simulink model "simple_streaming_txrx"  (Simulink 6.6)
settings: Solver=ode45  StartTime=0.0  StopTime=inf  RelTol=1e-3
InitFcn:
  | simple_streaming_init
StartFcn:
  | simple_streaming_init
undefined symbols (not defined in the file): dmf, gcbh, get, modConstellation_qam16, modConstellation_qam64, modConstellation_qpsk, rcosfir, symbolRomLen, txLSFR_initValues, txLSFR_polynomials, viqAvgLen, xlBlockLoadCallback, xlGetSimulinkPeriod
libraries: xbsIndex_r4 x506, commchan3 x2, commsink2 x1
(part 4 of 5)

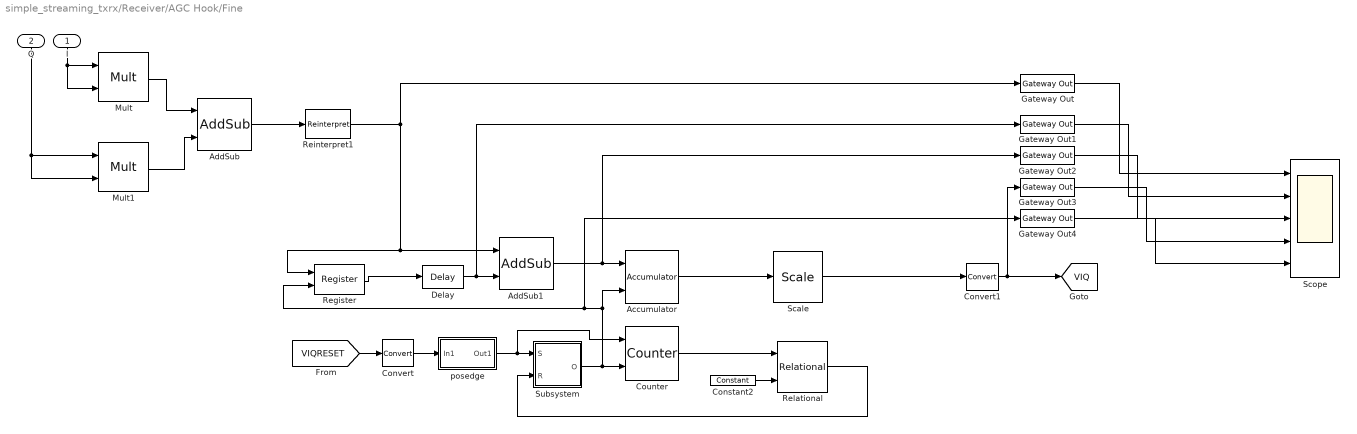
== system simple_streaming_txrx/Receiver/AGC Hook/Fine ==
  I : Inport  Orientation=down
  Q : Inport  Orientation=down  Port=2
  Accumulator : xbsIndex_r4/Accumulator  operation=Add  n_bits=30+ceil(log2(viqAvgLen))  overflow=Flag as error  scale=1  rst=on  hasbypass=off  en=off  dbl_ovrd=off  use_behavioral_HDL=on  block_type=accum
      settings: infoedit="Adder or subtractor-based accumulator.   Output type and binary point position match the input.<P><P>Hardware notes: When \"Reinitialize with input 'b' on reset\" is selected, the accumulator is forced to run at the system rate even if the input 'b' is running at a slower rate."  block_version=10.1.2
  AddSub : xbsIndex_r4/AddSub  mode=Addition  use_carryin=off  use_carryout=off  en=off  latency=0  precision=Full  arith_type=Unsigned  n_bits=16  bin_pt=14  quantization=Truncate  overflow=Wrap  dbl_ovrd=off  use_behavioral_HDL=off  pipelined=off  use_rpm=on  block_type=addsub
      settings: xl_area=[17 0 0 32 0 0 0]  block_version=10.1.2
  AddSub1 : xbsIndex_r4/AddSub  mode=Subtraction  use_carryin=off  use_carryout=off  en=off  latency=0  precision=Full  arith_type="Signed  (2's comp)"  n_bits=32  bin_pt=0  quantization=Truncate  overflow=Wrap  dbl_ovrd=off  use_behavioral_HDL=off  pipelined=off  use_rpm=on  block_type=addsub
      settings: block_version=10.1.2
  Constant2 : xbsIndex_r4/Constant  arith_type=Unsigned  const=viqAvgLen+2  n_bits=ceil(log2(viqAvgLen+1))  bin_pt=0  explicit_period=off  period=1  equ=P=C  opselect=C  inp2=PCIN>>17  opr=+  inp1=P  carry=CIN  dbl_ovrd=off  block_type=constant
      settings: block_version=10.1.2
  Convert : xbsIndex_r4/Convert  arith_type=Boolean  n_bits=16  bin_pt=14  quantization=Truncate  overflow=Wrap  latency=0  dbl_ovrd=off  pipeline=off  block_type=convert
      settings: block_version=10.1.2
  Convert1 : xbsIndex_r4/Convert  arith_type=Unsigned  n_bits=32  bin_pt=0  quantization=Truncate  overflow=Wrap  latency=0  dbl_ovrd=off  pipeline=off  block_type=convert
      settings: block_version=10.1.2
  Counter : xbsIndex_r4/Counter  cnt_type=Free Running  cnt_to=Inf  operation=Up  start_count=0  cnt_by_val=1  arith_type=Unsigned  n_bits=ceil(log2(viqAvgLen+1))  bin_pt=0  load_pin=off  rst=on  en=on  explicit_period=on  period=1/8  dbl_ovrd=off  use_behavioral_HDL=off  use_rpm=off  block_type=counter
      settings: block_version=10.1.2
  Delay : xbsIndex_r4/Delay  en=off  latency=viqAvgLen  dbl_ovrd=off  reg_retiming=off  block_type=delay
      settings: block_version=10.1.2
  Gateway Out{,1..4} (5 alike) : xbsIndex_r4/Gateway Out  hdl_port=off  timing_constraint=None  locs_specified=off  LOCs={}  block_type=gatewayout
      settings: infoedit="Gateway out block.  Converts Xilinx fixed point inputs into ouputs of type Simulink integer, double, or fixed point.<P><P>Hardware notes:  In hardware these blocks become top level output ports or are discarded, depending on how they are configured."  block_version=10.1.2
  Mult : xbsIndex_r4/Mult  precision=Full  arith_type=Unsigned  n_bits=32  bin_pt=32  quantization=Truncate  overflow=Saturate  en=off  latency=3  dbl_ovrd=off  use_behavioral_HDL=off  use_embedded=on  opt=Speed  optimum_pipeline=off  pipeline=on  use_rpm=on  placement_style=Triangular  block_type=mult
      settings: infoedit=Hardware notes: To use the internal pipeline stage of the dedicated multiplier you must select 'Pipeline for maximum performance'.  xl_area=[31 62 0 30 0 1 0]  block_version=10.1.2
  Mult1 : xbsIndex_r4/Mult  precision=Full  arith_type=Unsigned  n_bits=32  bin_pt=32  quantization=Truncate  overflow=Saturate  en=off  latency=3  dbl_ovrd=off  use_behavioral_HDL=off  use_embedded=on  opt=Speed  optimum_pipeline=off  pipeline=on  use_rpm=on  placement_style=Triangular  block_type=mult
      settings: infoedit=Hardware notes: To use the internal pipeline stage of the dedicated multiplier you must select 'Pipeline for maximum performance'.  xl_area=[31 62 0 30 0 1 0]  block_version=10.1.2
  Register : xbsIndex_r4/Register  init=0  rst=on  en=off  dbl_ovrd=off  block_type=register
      settings: block_version=10.1.2
  Reinterpret1 : xbsIndex_r4/Reinterpret  force_arith_type=on  arith_type=Unsigned  force_bin_pt=on  bin_pt=0  block_type=reinterpret
      settings: infoedit="Changes signal type without altering the binary representation.   You can changed the signal between signed and unsigned, and relocate the binary point.<P><P>Hardware notes: In hardware this block costs nothing.<P><P>Example:  Suppose the input is 6 bits wide, signed, with 2 fractional bits, and the output is forced to unsigned with 0 fractional bits.  Then an input of -2.0 (1110.00 in binary 2's complement) becomes an output of 56 (111000 in binary)."  block_version=10.1.2
  Relational : xbsIndex_r4/Relational  mode=a=b  en=off  latency=1  dbl_ovrd=off  block_type=relational
      settings: block_version=10.1.2
  Scale : xbsIndex_r4/Scale  scale_factor=-ceil(log2(viqAvgLen))  dbl_ovrd=off  block_type=scale
      settings: infoedit=Scales input by a power of two by adjusting the binary point position.<P><P>Hardware notes: In hardware this block costs nothing.  block_version=10.1.2
  Scope : Scope  NumInputPorts=5
      settings: YMin=0~0~-1.5e+006~1.06e+006~-1  YMax=2.75e+006~3e+006~2.5e+006~1.145e+006~1
  Subsystem : Subsystem
  posedge : Subsystem
  tag scope: VIQ=global
  wires:
  Mult1/1 -> AddSub/2
  Mult/1 -> AddSub/1
  I/1 -> Mult/1, Mult/2
  Q/1 -> Mult1/1, Mult1/2
  [VIQRESET] -> Convert/1
  posedge/1(Out1) -> Counter/1, Subsystem/1(S)
  Subsystem/1(O) -> Counter/2, Accumulator/2, Register/2, Gateway Out4/1
  Constant2/1 -> Relational/2
  Counter/1 -> Relational/1
  Relational/1 -> Subsystem/2(R)
  Accumulator/1 -> Scale/1
  Delay/1 -> AddSub1/2, Gateway Out1/1
  AddSub/1 -> Reinterpret1/1
  AddSub1/1 -> Accumulator/1, Gateway Out2/1
  Convert/1 -> posedge/1(In1)
  Convert1/1 -> [VIQ], Gateway Out3/1
  Reinterpret1/1 -> Gateway Out/1, AddSub1/1, Register/1
  Scale/1 -> Convert1/1
  Gateway Out/1 -> Scope/1
  Gateway Out1/1 -> Scope/2
  Gateway Out2/1 -> Scope/3
  Gateway Out3/1 -> Scope/4
  Gateway Out4/1 -> Scope/5
  Register/1 -> Delay/1

== system simple_streaming_txrx/Receiver/Carrier Recovery/2nd Order Filter ==
  Phase Error : Inport
  Reset : Inport  Port=2
  AddSub1 : xbsIndex_r4/AddSub  mode=Addition  use_carryin=off  use_carryout=off  en=off  latency=0  precision=Full  arith_type="Signed  (2's comp)"  n_bits=8  bin_pt=2  quantization=Truncate  overflow=Flag as error  dbl_ovrd=off  use_behavioral_HDL=on  pipelined=off  use_rpm=on  block_type=addsub
      settings: xl_area=[19 0 0 36 0 0 0]  block_version=10.1
  AddSub2 : xbsIndex_r4/AddSub  mode=Addition  use_carryin=off  use_carryout=off  en=off  latency=0  precision=User Defined  arith_type="Signed  (2's comp)"  n_bits=35  bin_pt=34  quantization=Truncate  overflow=Flag as error  dbl_ovrd=off  use_behavioral_HDL=on  pipelined=off  use_rpm=on  block_type=addsub
      settings: xl_area=[19 0 0 36 0 0 0]  block_version=10.1
  Delay1 : xbsIndex_r4/Delay  en=off  latency=1  dbl_ovrd=off  reg_retiming=off  block_type=delay
      settings: xl_area=[18 35 0 0 0 0 0]  block_version=10.1
  Delay2 : xbsIndex_r4/Delay  en=off  latency=1  dbl_ovrd=off  reg_retiming=off  block_type=delay
      settings: xl_area=[18 35 0 0 0 0 0]  block_version=10.1
  Mult1 : xbsIndex_r4/Mult  precision=User Defined  arith_type="Signed  (2's comp)"  n_bits=35  bin_pt=34  quantization=Truncate  overflow=Flag as error  en=off  latency=3  dbl_ovrd=off  use_behavioral_HDL=off  use_embedded=on  opt=Speed  optimum_pipeline=off  pipeline=on  use_rpm=on  placement_style=Rectangular shape  block_type=mult
      settings: infoedit=Hardware notes: To use the internal pipeline stage of the dedicated multiplier you must select 'Pipeline for maximum performance'.  xl_area=[89 143 0 153 0 4 0]  block_version=10.1
  Mult2 : xbsIndex_r4/Mult  precision=User Defined  arith_type="Signed  (2's comp)"  n_bits=35  bin_pt=34  quantization=Truncate  overflow=Flag as error  en=off  latency=3  dbl_ovrd=off  use_behavioral_HDL=off  use_embedded=on  opt=Speed  optimum_pipeline=off  pipeline=on  use_rpm=on  placement_style=Rectangular shape  block_type=mult
      settings: infoedit=Hardware notes: To use the internal pipeline stage of the dedicated multiplier you must select 'Pipeline for maximum performance'.  xl_area=[89 143 0 153 0 4 0]  block_version=10.1
  Register1 : xbsIndex_r4/Register  init=0  rst=on  en=off  dbl_ovrd=off  block_type=register
      settings: xl_area=[18 36 0 0 0 0 0]  block_version=10.1
  Register2 : xbsIndex_r4/Register  Orientation=left  init=0  rst=on  en=off  dbl_ovrd=off  block_type=register
      settings: xl_area=[18 35 0 0 0 0 0]  block_version=10.1
  Phase Inc : Outport
  wires:
  Delay2/1 -> AddSub1/1
  Register2/1 -> AddSub2/2
  AddSub2/1 -> Delay1/1, Register2/1
  Mult1/1 -> AddSub2/1
  Mult2/1 -> Delay2/1
  AddSub1/1 -> Register1/1
  Reset/1 -> Register1/2, Register2/2
  Register1/1 -> Phase Inc/1
  Phase Error/1 -> Mult2/2, Mult1/1
  [CFO_KI] -> Mult1/2
  [CFO_KP] -> Mult2/1
  Delay1/1 -> AddSub1/2

== system simple_streaming_txrx/Receiver/Carrier Recovery/Phase Error Detector ==
  I : Inport
  Q : Inport  Port=2
  AddSub : xbsIndex_r4/AddSub  mode=Subtraction  use_carryin=off  use_carryout=off  en=off  latency=0  precision=Full  arith_type="Signed  (2's comp)"  n_bits=16  bin_pt=13  quantization=Truncate  overflow=Wrap  dbl_ovrd=off  use_behavioral_HDL=on  pipelined=off  use_rpm=on  block_type=addsub
      settings: xl_area=[10 0 0 19 0 0 0]  block_version=10.1
  Mult : xbsIndex_r4/Mult  precision=Full  arith_type="Signed  (2's comp)"  n_bits=16  bin_pt=14  quantization=Truncate  overflow=Wrap  en=off  latency=1  dbl_ovrd=off  use_behavioral_HDL=off  use_embedded=on  opt=Speed  optimum_pipeline=off  pipeline=on  use_rpm=on  placement_style=Rectangular shape  block_type=mult
      settings: infoedit=Hardware notes: To use the internal pipeline stage of the dedicated multiplier you must select 'Pipeline for maximum performance'.  xl_area=[9 0 0 18 0 1 0]  block_version=10.1
  Mult1 : xbsIndex_r4/Mult  precision=Full  arith_type="Signed  (2's comp)"  n_bits=16  bin_pt=14  quantization=Truncate  overflow=Wrap  en=off  latency=1  dbl_ovrd=off  use_behavioral_HDL=off  use_embedded=on  opt=Speed  optimum_pipeline=off  pipeline=on  use_rpm=on  placement_style=Rectangular shape  block_type=mult
      settings: infoedit=Hardware notes: To use the internal pipeline stage of the dedicated multiplier you must select 'Pipeline for maximum performance'.  xl_area=[9 0 0 18 0 1 0]  block_version=10.1
  Threshold : xbsIndex_r4/Threshold  en=off  latency=0  dbl_ovrd=off  block_type=sgn
      settings: infoedit="Presents -1 as output if input is negative; otherwise presents 1.  Output is a two bit signed number."  xl_area=[0 0 0 0 0 0 0]  block_version=10.1
  Threshold1 : xbsIndex_r4/Threshold  en=off  latency=0  dbl_ovrd=off  block_type=sgn
      settings: infoedit="Presents -1 as output if input is negative; otherwise presents 1.  Output is a two bit signed number."  xl_area=[0 0 0 0 0 0 0]  block_version=10.1
  Err : Outport
  wires:
  Threshold1/1 -> Mult1/1
  Threshold/1 -> Mult/1
  Mult/1 -> AddSub/1
  Mult1/1 -> AddSub/2
  I/1 -> Mult1/2, Threshold/1
  Q/1 -> Mult/2, Threshold1/1
  AddSub/1 -> Err/1

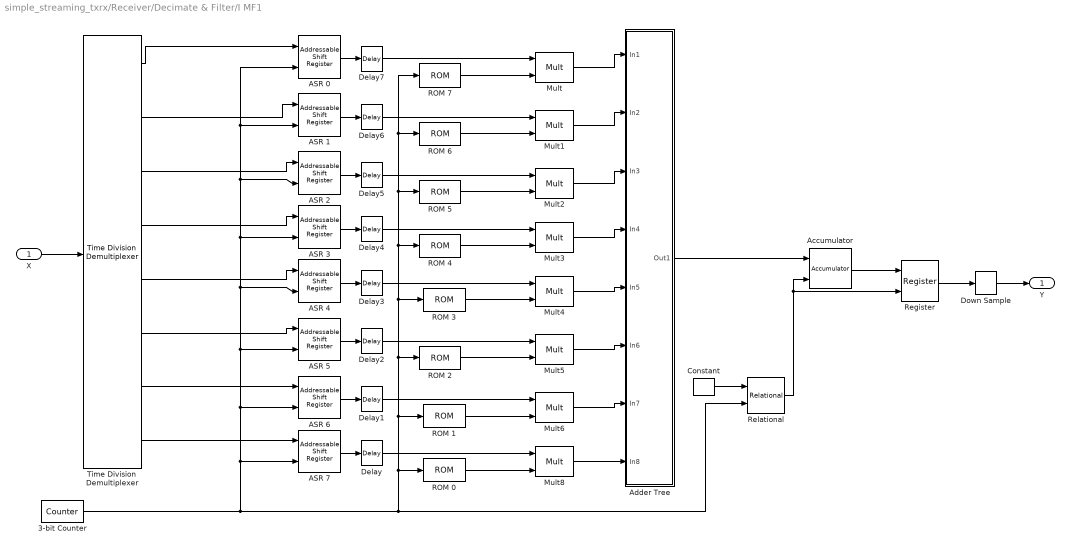
== system simple_streaming_txrx/Receiver/Decimate & Filter/I MF1 ==
  X : Inport
  3-bit Counter : xbsIndex_r4/Counter  cnt_type=Free Running  cnt_to=Inf  operation=Up  start_count=0  cnt_by_val=1  arith_type=Unsigned  n_bits=3  bin_pt=0  load_pin=off  rst=off  en=off  explicit_period=off  period=data_samplePeriod  dbl_ovrd=off  use_behavioral_HDL=off  use_rpm=on  block_type=counter
      settings: xl_area=[3 3 0 3 0 0 0]  block_version=10.1
  ASR {0..7} (8 alike) : xbsIndex_r4/Addressable Shift Register  infer_latency=on  depth=2  initVector=[0]  en=off  dbl_ovrd=off  use_behavioral_HDL=off  use_rpm=on  block_type=addrsr
      settings: infoedit="Delay of configurable length.  Any element in the delay line can be addressed and driven onto the output port.<br><br>Hardware notes: Implemented using SRL16s.  If Virtex-4, Virtex-II or Spartan-3 devices are used, multiple SRLC16s are cascaded together."  xl_area=[9 0 0 18 0 0 0]  block_version=10.1
  Accumulator : xbsIndex_r4/Accumulator  operation=Add  n_bits=add_prec  overflow=Wrap  scale=1  rst=on  hasbypass=on  en=off  dbl_ovrd=off  use_behavioral_HDL=on  block_type=accum
      settings: infoedit="Adder or subtractor-based accumulator.   Output type and binary point position match the input.<P><P>Hardware notes: When \"Reinitialize with input 'b' on reset\" is selected, the accumulator is forced to run at the system rate even if the input 'b' is running at a slower rate."  xl_area=[9 17 0 16 0 0 0]  block_version=10.1
  Adder Tree : Subsystem
  Constant : xbsIndex_r4/Constant  arith_type=Unsigned  const=3  n_bits=3  bin_pt=0  explicit_period=on  period=data_samplePeriod  equ=P=C  opselect=C  inp2=PCIN>>17  opr=+  inp1=P  carry=CIN  dbl_ovrd=off  block_type=constant
      settings: block_version=10.1
  Delay{,1..7} (8 alike) : xbsIndex_r4/Delay  en=off  latency=1  dbl_ovrd=off  reg_retiming=off  block_type=delay
      settings: xl_area=[9 18 0 0 0 0 0]  block_version=10.1
  Down Sample : xbsIndex_r4/Down Sample  sample_ratio=8  sample_phase=First Value of Frame  en=off  latency=0  dbl_ovrd=off  block_type=dsamp
      settings: xl_area=[17 17 0 16 0 0 0]  block_version=10.1
  Mult{,1..6,8} (8 alike) : xbsIndex_r4/Mult  precision=User Defined  arith_type="Signed  (2's comp)"  n_bits=mult_prec  bin_pt=mult_bp  quantization=Truncate  overflow=Flag as error  en=off  latency=multLatency  dbl_ovrd=off  use_behavioral_HDL=off  use_embedded=on  opt=Speed  optimum_pipeline=off  pipeline=on  use_rpm=on  placement_style=Rectangular shape  block_type=mult
      settings: infoedit=Hardware notes: To use the internal pipeline stage of the dedicated multiplier you must select 'Pipeline for maximum performance'.  xl_area=[9 -13 0 18 0 1 0]  block_version=10.1
  ROM 0 : xbsIndex_r4/ROM  depth=polyphaseBranches  initVector=h(1:subFilterLength)  distributed_mem=Distributed memory  rst=off  init_reg=0  en=off  latency=1  arith_type="Signed  (2's comp)"  n_bits=coeff_prec  bin_pt=coeff_bp  dbl_ovrd=off  optimize=Area  use_rpm=off  block_type=sprom
      settings: xl_area=[7 14 0 13 0 0 0]  block_version=10.1
  ROM 1 : xbsIndex_r4/ROM  depth=polyphaseBranches  initVector=h(1*subFilterLength+1:2*subFilterLength)  distributed_mem=Distributed memory  rst=off  init_reg=0  en=off  latency=1  arith_type="Signed  (2's comp)"  n_bits=coeff_prec  bin_pt=coeff_bp  dbl_ovrd=off  optimize=Area  use_rpm=off  block_type=sprom
      settings: xl_area=[7 14 0 14 0 0 0]  block_version=10.1
  ROM 2 : xbsIndex_r4/ROM  depth=polyphaseBranches  initVector=h(2*subFilterLength+1:3*subFilterLength)  distributed_mem=Distributed memory  rst=off  init_reg=0  en=off  latency=1  arith_type="Signed  (2's comp)"  n_bits=coeff_prec  bin_pt=coeff_bp  dbl_ovrd=off  optimize=Area  use_rpm=off  block_type=sprom
      settings: xl_area=[7 14 0 14 0 0 0]  block_version=10.1
  ROM 3 : xbsIndex_r4/ROM  depth=polyphaseBranches  initVector=h(3*subFilterLength+1:4*subFilterLength)  distributed_mem=Distributed memory  rst=off  init_reg=0  en=off  latency=1  arith_type="Signed  (2's comp)"  n_bits=coeff_prec  bin_pt=coeff_bp  dbl_ovrd=off  optimize=Area  use_rpm=off  block_type=sprom
      settings: xl_area=[7 14 0 14 0 0 0]  block_version=10.1
  ROM 4 : xbsIndex_r4/ROM  depth=polyphaseBranches  initVector=h(4*subFilterLength+1:5*subFilterLength)  distributed_mem=Distributed memory  rst=off  init_reg=0  en=off  latency=1  arith_type="Signed  (2's comp)"  n_bits=coeff_prec  bin_pt=coeff_bp  dbl_ovrd=off  optimize=Area  use_rpm=off  block_type=sprom
      settings: xl_area=[7 14 0 14 0 0 0]  block_version=10.1
  ROM 5 : xbsIndex_r4/ROM  depth=polyphaseBranches  initVector=h(5*subFilterLength+1:6*subFilterLength)  distributed_mem=Distributed memory  rst=off  init_reg=0  en=off  latency=1  arith_type="Signed  (2's comp)"  n_bits=coeff_prec  bin_pt=coeff_bp  dbl_ovrd=off  optimize=Area  use_rpm=off  block_type=sprom
      settings: xl_area=[7 14 0 14 0 0 0]  block_version=10.1
  ROM 6 : xbsIndex_r4/ROM  depth=polyphaseBranches  initVector=h(6*subFilterLength+1:7*subFilterLength)  distributed_mem=Distributed memory  rst=off  init_reg=0  en=off  latency=1  arith_type="Signed  (2's comp)"  n_bits=coeff_prec  bin_pt=coeff_bp  dbl_ovrd=off  optimize=Area  use_rpm=off  block_type=sprom
      settings: xl_area=[7 14 0 14 0 0 0]  block_version=10.1
  ROM 7 : xbsIndex_r4/ROM  depth=polyphaseBranches  initVector=h(7*subFilterLength+1:8*subFilterLength)  distributed_mem=Distributed memory  rst=off  init_reg=0  en=off  latency=1  arith_type="Signed  (2's comp)"  n_bits=coeff_prec  bin_pt=coeff_bp  dbl_ovrd=off  optimize=Area  use_rpm=off  block_type=sprom
      settings: xl_area=[7 14 0 14 0 0 0]  block_version=10.1
  Register : xbsIndex_r4/Register  init=0  rst=off  en=on  dbl_ovrd=off  block_type=register
      settings: xl_area=[8 16 0 0 0 0 0]  block_version=10.1
  Relational : xbsIndex_r4/Relational  mode=a=b  en=off  latency=0  dbl_ovrd=off  block_type=relational
      settings: xl_area=[1 0 0 2 0 0 0]  block_version=10.1
  Time Division Demultiplexer : xbsIndex_r4/Time Division Demultiplexer  frame_pattern=ones(1,8)  impl_style=Multiple Channel  vin=off  dbl_ovrd=off  explicit_period=off  period=1  block_type=tdd
      settings: infoedit=Samples presented at the input are selected and down-sampled according to the frame sampling pattern specified. The sampled input is presented either as a single or multiple channel at the output.  xl_area=[135 270 0 0 0 0 0]  block_version=10.1
  Y : Outport
  wires:
  3-bit Counter/1 -> ROM 6/1, ROM 7/1, ROM 5/1, ROM 4/1, ROM 3/1, ROM 2/1, ROM 1/1, ROM 0/1, Relational/2, ASR 7/2, ASR 6/2, ASR 5/2, ASR 4/2, ASR 3/2, ASR 2/2, ASR 0/2, ASR 1/2
  ASR 7/1 -> Delay/1
  ASR 6/1 -> Delay1/1
  ASR 5/1 -> Delay2/1
  ASR 4/1 -> Delay3/1
  ASR 3/1 -> Delay4/1
  ASR 2/1 -> Delay5/1
  ASR 1/1 -> Delay6/1
  ASR 0/1 -> Delay7/1
  Mult8/1 -> Adder Tree/8(In8)
  Mult6/1 -> Adder Tree/7(In7)
  Mult5/1 -> Adder Tree/6(In6)
  Mult4/1 -> Adder Tree/5(In5)
  Mult3/1 -> Adder Tree/4(In4)
  Mult2/1 -> Adder Tree/3(In3)
  Mult1/1 -> Adder Tree/2(In2)
  Mult/1 -> Adder Tree/1(In1)
  ROM 0/1 -> Mult8/2
  ROM 1/1 -> Mult6/2
  ROM 2/1 -> Mult5/2
  ROM 3/1 -> Mult4/2
  ROM 4/1 -> Mult3/2
  ROM 5/1 -> Mult2/2
  ROM 6/1 -> Mult1/2
  ROM 7/1 -> Mult/2
  Accumulator/1 -> Register/1
  Constant/1 -> Relational/1
  Relational/1 -> Accumulator/2, Register/2
  Down Sample/1 -> Y/1
  Register/1 -> Down Sample/1
  Adder Tree/1(Out1) -> Accumulator/1
  X/1 -> Time Division Demultiplexer/1
  Time Division Demultiplexer/1 -> ASR 0/1
  Time Division Demultiplexer/2 -> ASR 1/1
  Time Division Demultiplexer/3 -> ASR 2/1
  Time Division Demultiplexer/4 -> ASR 3/1
  Time Division Demultiplexer/5 -> ASR 4/1
  Time Division Demultiplexer/6 -> ASR 5/1
  Time Division Demultiplexer/7 -> ASR 6/1
  Time Division Demultiplexer/8 -> ASR 7/1
  Delay/1 -> Mult8/1
  Delay1/1 -> Mult6/1
  Delay2/1 -> Mult5/1
  Delay3/1 -> Mult4/1
  Delay4/1 -> Mult3/1
  Delay5/1 -> Mult2/1
  Delay6/1 -> Mult1/1
  Delay7/1 -> Mult/1

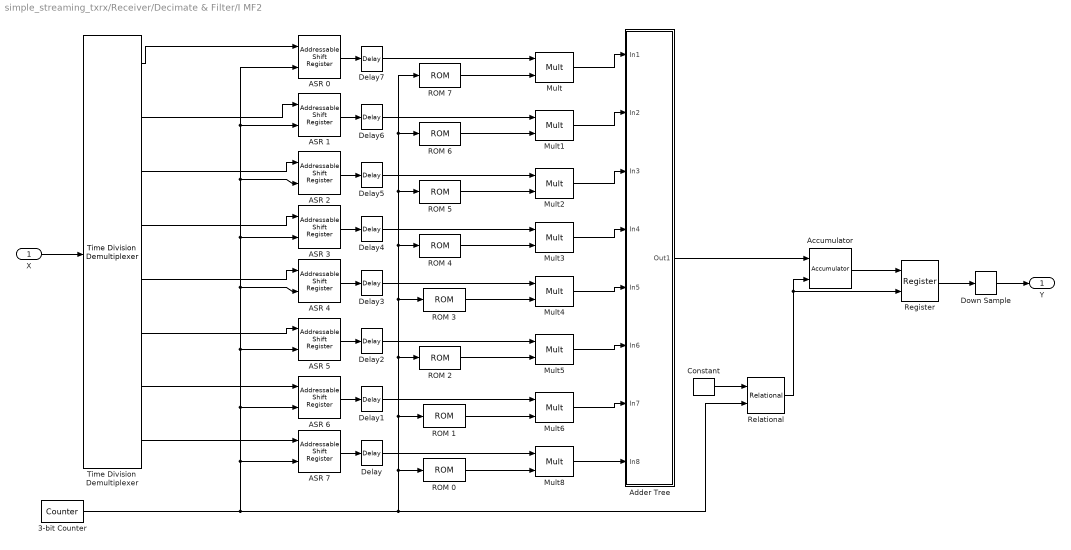
== system simple_streaming_txrx/Receiver/Decimate & Filter/I MF2 ==
  X : Inport
  3-bit Counter : xbsIndex_r4/Counter  cnt_type=Free Running  cnt_to=Inf  operation=Up  start_count=0  cnt_by_val=1  arith_type=Unsigned  n_bits=3  bin_pt=0  load_pin=off  rst=off  en=off  explicit_period=off  period=data_samplePeriod  dbl_ovrd=off  use_behavioral_HDL=off  use_rpm=on  block_type=counter
      settings: xl_area=[3 3 0 3 0 0 0]  block_version=10.1
  ASR {0..7} (8 alike) : xbsIndex_r4/Addressable Shift Register  infer_latency=on  depth=2  initVector=[0]  en=off  dbl_ovrd=off  use_behavioral_HDL=off  use_rpm=on  block_type=addrsr
      settings: infoedit="Delay of configurable length.  Any element in the delay line can be addressed and driven onto the output port.<br><br>Hardware notes: Implemented using SRL16s.  If Virtex-4, Virtex-II or Spartan-3 devices are used, multiple SRLC16s are cascaded together."  xl_area=[9 0 0 18 0 0 0]  block_version=10.1
  Accumulator : xbsIndex_r4/Accumulator  operation=Add  n_bits=add_prec  overflow=Wrap  scale=1  rst=on  hasbypass=on  en=off  dbl_ovrd=off  use_behavioral_HDL=on  block_type=accum
      settings: infoedit="Adder or subtractor-based accumulator.   Output type and binary point position match the input.<P><P>Hardware notes: When \"Reinitialize with input 'b' on reset\" is selected, the accumulator is forced to run at the system rate even if the input 'b' is running at a slower rate."  xl_area=[9 17 0 16 0 0 0]  block_version=10.1
  Adder Tree : Subsystem
  Constant : xbsIndex_r4/Constant  arith_type=Unsigned  const=3  n_bits=3  bin_pt=0  explicit_period=on  period=data_samplePeriod  equ=P=C  opselect=C  inp2=PCIN>>17  opr=+  inp1=P  carry=CIN  dbl_ovrd=off  block_type=constant
      settings: block_version=10.1
  Delay{,1..7} (8 alike) : xbsIndex_r4/Delay  en=off  latency=1  dbl_ovrd=off  reg_retiming=off  block_type=delay
      settings: xl_area=[9 18 0 0 0 0 0]  block_version=10.1
  Down Sample : xbsIndex_r4/Down Sample  sample_ratio=8  sample_phase=First Value of Frame  en=off  latency=0  dbl_ovrd=off  block_type=dsamp
      settings: xl_area=[17 17 0 16 0 0 0]  block_version=10.1
  Mult{,1..6,8} (8 alike) : xbsIndex_r4/Mult  precision=User Defined  arith_type="Signed  (2's comp)"  n_bits=mult_prec  bin_pt=mult_bp  quantization=Truncate  overflow=Flag as error  en=off  latency=multLatency  dbl_ovrd=off  use_behavioral_HDL=off  use_embedded=on  opt=Speed  optimum_pipeline=off  pipeline=on  use_rpm=on  placement_style=Rectangular shape  block_type=mult
      settings: infoedit=Hardware notes: To use the internal pipeline stage of the dedicated multiplier you must select 'Pipeline for maximum performance'.  xl_area=[9 -13 0 18 0 1 0]  block_version=10.1
  ROM 0 : xbsIndex_r4/ROM  depth=polyphaseBranches  initVector=h(1:subFilterLength)  distributed_mem=Distributed memory  rst=off  init_reg=0  en=off  latency=1  arith_type="Signed  (2's comp)"  n_bits=coeff_prec  bin_pt=coeff_bp  dbl_ovrd=off  optimize=Area  use_rpm=off  block_type=sprom
      settings: xl_area=[7 14 0 13 0 0 0]  block_version=10.1
  ROM 1 : xbsIndex_r4/ROM  depth=polyphaseBranches  initVector=h(1*subFilterLength+1:2*subFilterLength)  distributed_mem=Distributed memory  rst=off  init_reg=0  en=off  latency=1  arith_type="Signed  (2's comp)"  n_bits=coeff_prec  bin_pt=coeff_bp  dbl_ovrd=off  optimize=Area  use_rpm=off  block_type=sprom
      settings: xl_area=[7 14 0 14 0 0 0]  block_version=10.1
  ROM 2 : xbsIndex_r4/ROM  depth=polyphaseBranches  initVector=h(2*subFilterLength+1:3*subFilterLength)  distributed_mem=Distributed memory  rst=off  init_reg=0  en=off  latency=1  arith_type="Signed  (2's comp)"  n_bits=coeff_prec  bin_pt=coeff_bp  dbl_ovrd=off  optimize=Area  use_rpm=off  block_type=sprom
      settings: xl_area=[7 14 0 14 0 0 0]  block_version=10.1
  ROM 3 : xbsIndex_r4/ROM  depth=polyphaseBranches  initVector=h(3*subFilterLength+1:4*subFilterLength)  distributed_mem=Distributed memory  rst=off  init_reg=0  en=off  latency=1  arith_type="Signed  (2's comp)"  n_bits=coeff_prec  bin_pt=coeff_bp  dbl_ovrd=off  optimize=Area  use_rpm=off  block_type=sprom
      settings: xl_area=[7 14 0 14 0 0 0]  block_version=10.1
  ROM 4 : xbsIndex_r4/ROM  depth=polyphaseBranches  initVector=h(4*subFilterLength+1:5*subFilterLength)  distributed_mem=Distributed memory  rst=off  init_reg=0  en=off  latency=1  arith_type="Signed  (2's comp)"  n_bits=coeff_prec  bin_pt=coeff_bp  dbl_ovrd=off  optimize=Area  use_rpm=off  block_type=sprom
      settings: xl_area=[7 14 0 14 0 0 0]  block_version=10.1
  ROM 5 : xbsIndex_r4/ROM  depth=polyphaseBranches  initVector=h(5*subFilterLength+1:6*subFilterLength)  distributed_mem=Distributed memory  rst=off  init_reg=0  en=off  latency=1  arith_type="Signed  (2's comp)"  n_bits=coeff_prec  bin_pt=coeff_bp  dbl_ovrd=off  optimize=Area  use_rpm=off  block_type=sprom
      settings: xl_area=[7 14 0 14 0 0 0]  block_version=10.1
  ROM 6 : xbsIndex_r4/ROM  depth=polyphaseBranches  initVector=h(6*subFilterLength+1:7*subFilterLength)  distributed_mem=Distributed memory  rst=off  init_reg=0  en=off  latency=1  arith_type="Signed  (2's comp)"  n_bits=coeff_prec  bin_pt=coeff_bp  dbl_ovrd=off  optimize=Area  use_rpm=off  block_type=sprom
      settings: xl_area=[7 14 0 14 0 0 0]  block_version=10.1
  ROM 7 : xbsIndex_r4/ROM  depth=polyphaseBranches  initVector=h(7*subFilterLength+1:8*subFilterLength)  distributed_mem=Distributed memory  rst=off  init_reg=0  en=off  latency=1  arith_type="Signed  (2's comp)"  n_bits=coeff_prec  bin_pt=coeff_bp  dbl_ovrd=off  optimize=Area  use_rpm=off  block_type=sprom
      settings: xl_area=[7 14 0 14 0 0 0]  block_version=10.1
  Register : xbsIndex_r4/Register  init=0  rst=off  en=on  dbl_ovrd=off  block_type=register
      settings: xl_area=[8 16 0 0 0 0 0]  block_version=10.1
  Relational : xbsIndex_r4/Relational  mode=a=b  en=off  latency=0  dbl_ovrd=off  block_type=relational
      settings: xl_area=[1 0 0 2 0 0 0]  block_version=10.1
  Time Division Demultiplexer : xbsIndex_r4/Time Division Demultiplexer  frame_pattern=ones(1,8)  impl_style=Multiple Channel  vin=off  dbl_ovrd=off  explicit_period=off  period=1  block_type=tdd
      settings: infoedit=Samples presented at the input are selected and down-sampled according to the frame sampling pattern specified. The sampled input is presented either as a single or multiple channel at the output.  xl_area=[135 270 0 0 0 0 0]  block_version=10.1
  Y : Outport
  wires:
  Delay7/1 -> Mult/1
  Delay6/1 -> Mult1/1
  Delay5/1 -> Mult2/1
  Delay4/1 -> Mult3/1
  Delay3/1 -> Mult4/1
  Delay2/1 -> Mult5/1
  Delay1/1 -> Mult6/1
  Delay/1 -> Mult8/1
  Time Division Demultiplexer/8 -> ASR 7/1
  Time Division Demultiplexer/7 -> ASR 6/1
  Time Division Demultiplexer/6 -> ASR 5/1
  Time Division Demultiplexer/5 -> ASR 4/1
  Time Division Demultiplexer/4 -> ASR 3/1
  Time Division Demultiplexer/3 -> ASR 2/1
  Time Division Demultiplexer/2 -> ASR 1/1
  Time Division Demultiplexer/1 -> ASR 0/1
  X/1 -> Time Division Demultiplexer/1
  Adder Tree/1(Out1) -> Accumulator/1
  Register/1 -> Down Sample/1
  Down Sample/1 -> Y/1
  Relational/1 -> Register/2, Accumulator/2
  Constant/1 -> Relational/1
  Accumulator/1 -> Register/1
  ROM 7/1 -> Mult/2
  ROM 6/1 -> Mult1/2
  ROM 5/1 -> Mult2/2
  ROM 4/1 -> Mult3/2
  ROM 3/1 -> Mult4/2
  ROM 2/1 -> Mult5/2
  ROM 1/1 -> Mult6/2
  ROM 0/1 -> Mult8/2
  Mult/1 -> Adder Tree/1(In1)
  Mult1/1 -> Adder Tree/2(In2)
  Mult2/1 -> Adder Tree/3(In3)
  Mult3/1 -> Adder Tree/4(In4)
  Mult4/1 -> Adder Tree/5(In5)
  Mult5/1 -> Adder Tree/6(In6)
  Mult6/1 -> Adder Tree/7(In7)
  Mult8/1 -> Adder Tree/8(In8)
  ASR 0/1 -> Delay7/1
  ASR 1/1 -> Delay6/1
  ASR 2/1 -> Delay5/1
  ASR 3/1 -> Delay4/1
  ASR 4/1 -> Delay3/1
  ASR 5/1 -> Delay2/1
  ASR 6/1 -> Delay1/1
  ASR 7/1 -> Delay/1
  3-bit Counter/1 -> ASR 1/2, ASR 0/2, ASR 2/2, ASR 3/2, ASR 4/2, ASR 5/2, ASR 6/2, ASR 7/2, Relational/2, ROM 0/1, ROM 1/1, ROM 2/1, ROM 3/1, ROM 4/1, ROM 5/1, ROM 7/1, ROM 6/1

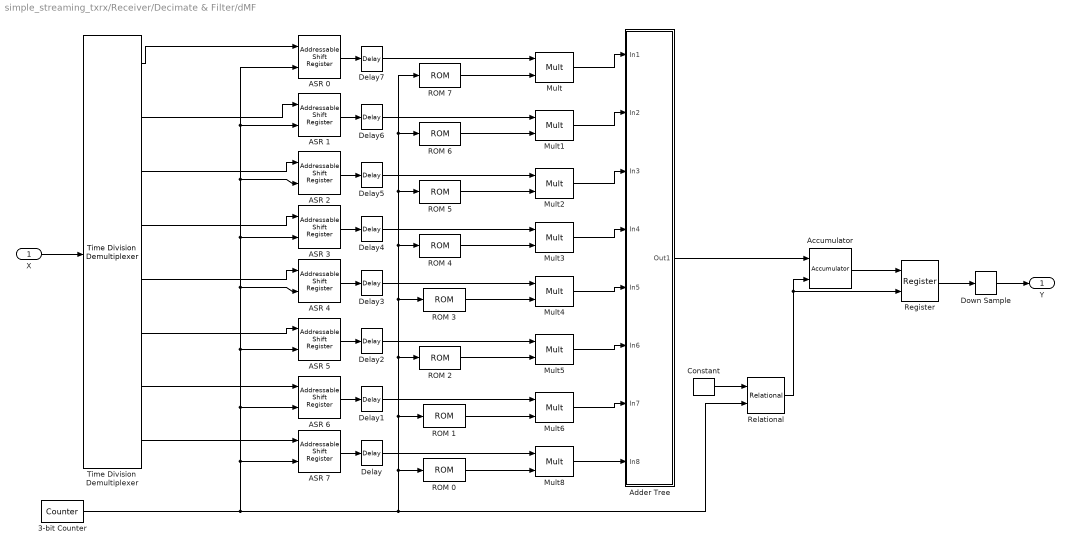
== system simple_streaming_txrx/Receiver/Decimate & Filter/dMF ==
  X : Inport
  3-bit Counter : xbsIndex_r4/Counter  cnt_type=Free Running  cnt_to=Inf  operation=Up  start_count=0  cnt_by_val=1  arith_type=Unsigned  n_bits=3  bin_pt=0  load_pin=off  rst=off  en=off  explicit_period=off  period=data_samplePeriod  dbl_ovrd=off  use_behavioral_HDL=off  use_rpm=on  block_type=counter
      settings: xl_area=[3 3 0 3 0 0 0]  block_version=10.1
  ASR {0..7} (8 alike) : xbsIndex_r4/Addressable Shift Register  infer_latency=on  depth=2  initVector=[0]  en=off  dbl_ovrd=off  use_behavioral_HDL=off  use_rpm=on  block_type=addrsr
      settings: infoedit="Delay of configurable length.  Any element in the delay line can be addressed and driven onto the output port.<br><br>Hardware notes: Implemented using SRL16s.  If Virtex-4, Virtex-II or Spartan-3 devices are used, multiple SRLC16s are cascaded together."  xl_area=[9 0 0 18 0 0 0]  block_version=10.1
  Accumulator : xbsIndex_r4/Accumulator  operation=Add  n_bits=add_prec  overflow=Wrap  scale=1  rst=on  hasbypass=on  en=off  dbl_ovrd=off  use_behavioral_HDL=on  block_type=accum
      settings: infoedit="Adder or subtractor-based accumulator.   Output type and binary point position match the input.<P><P>Hardware notes: When \"Reinitialize with input 'b' on reset\" is selected, the accumulator is forced to run at the system rate even if the input 'b' is running at a slower rate."  xl_area=[9 17 0 16 0 0 0]  block_version=10.1
  Adder Tree : Subsystem
  Constant : xbsIndex_r4/Constant  arith_type=Unsigned  const=3  n_bits=3  bin_pt=0  explicit_period=on  period=data_samplePeriod  equ=P=C  opselect=C  inp2=PCIN>>17  opr=+  inp1=P  carry=CIN  dbl_ovrd=off  block_type=constant
      settings: block_version=10.1
  Delay{,1..7} (8 alike) : xbsIndex_r4/Delay  en=off  latency=1  dbl_ovrd=off  reg_retiming=off  block_type=delay
      settings: xl_area=[9 18 0 0 0 0 0]  block_version=10.1
  Down Sample : xbsIndex_r4/Down Sample  sample_ratio=8  sample_phase=First Value of Frame  en=off  latency=0  dbl_ovrd=off  block_type=dsamp
      settings: xl_area=[17 17 0 16 0 0 0]  block_version=10.1
  Mult{,1..6,8} (8 alike) : xbsIndex_r4/Mult  precision=User Defined  arith_type="Signed  (2's comp)"  n_bits=mult_prec  bin_pt=mult_bp  quantization=Truncate  overflow=Flag as error  en=off  latency=multLatency  dbl_ovrd=off  use_behavioral_HDL=off  use_embedded=on  opt=Speed  optimum_pipeline=off  pipeline=on  use_rpm=on  placement_style=Rectangular shape  block_type=mult
      settings: infoedit=Hardware notes: To use the internal pipeline stage of the dedicated multiplier you must select 'Pipeline for maximum performance'.  xl_area=[9 -13 0 18 0 1 0]  block_version=10.1
  ROM 0 : xbsIndex_r4/ROM  depth=polyphaseBranches  initVector=h(1:subFilterLength)  distributed_mem=Distributed memory  rst=off  init_reg=0  en=off  latency=1  arith_type="Signed  (2's comp)"  n_bits=coeff_prec  bin_pt=coeff_bp  dbl_ovrd=off  optimize=Area  use_rpm=off  block_type=sprom
      settings: xl_area=[7 14 0 14 0 0 0]  block_version=10.1
  ROM 1 : xbsIndex_r4/ROM  depth=polyphaseBranches  initVector=h(1*subFilterLength+1:2*subFilterLength)  distributed_mem=Distributed memory  rst=off  init_reg=0  en=off  latency=1  arith_type="Signed  (2's comp)"  n_bits=coeff_prec  bin_pt=coeff_bp  dbl_ovrd=off  optimize=Area  use_rpm=off  block_type=sprom
      settings: xl_area=[7 14 0 14 0 0 0]  block_version=10.1
  ROM 2 : xbsIndex_r4/ROM  depth=polyphaseBranches  initVector=h(2*subFilterLength+1:3*subFilterLength)  distributed_mem=Distributed memory  rst=off  init_reg=0  en=off  latency=1  arith_type="Signed  (2's comp)"  n_bits=coeff_prec  bin_pt=coeff_bp  dbl_ovrd=off  optimize=Area  use_rpm=off  block_type=sprom
      settings: xl_area=[7 14 0 14 0 0 0]  block_version=10.1
  ROM 3 : xbsIndex_r4/ROM  depth=polyphaseBranches  initVector=h(3*subFilterLength+1:4*subFilterLength)  distributed_mem=Distributed memory  rst=off  init_reg=0  en=off  latency=1  arith_type="Signed  (2's comp)"  n_bits=coeff_prec  bin_pt=coeff_bp  dbl_ovrd=off  optimize=Area  use_rpm=off  block_type=sprom
      settings: xl_area=[7 14 0 14 0 0 0]  block_version=10.1
  ROM 4 : xbsIndex_r4/ROM  depth=polyphaseBranches  initVector=h(4*subFilterLength+1:5*subFilterLength)  distributed_mem=Distributed memory  rst=off  init_reg=0  en=off  latency=1  arith_type="Signed  (2's comp)"  n_bits=coeff_prec  bin_pt=coeff_bp  dbl_ovrd=off  optimize=Area  use_rpm=off  block_type=sprom
      settings: xl_area=[7 14 0 14 0 0 0]  block_version=10.1
  ROM 5 : xbsIndex_r4/ROM  depth=polyphaseBranches  initVector=h(5*subFilterLength+1:6*subFilterLength)  distributed_mem=Distributed memory  rst=off  init_reg=0  en=off  latency=1  arith_type="Signed  (2's comp)"  n_bits=coeff_prec  bin_pt=coeff_bp  dbl_ovrd=off  optimize=Area  use_rpm=off  block_type=sprom
      settings: xl_area=[7 14 0 14 0 0 0]  block_version=10.1
  ROM 6 : xbsIndex_r4/ROM  depth=polyphaseBranches  initVector=h(6*subFilterLength+1:7*subFilterLength)  distributed_mem=Distributed memory  rst=off  init_reg=0  en=off  latency=1  arith_type="Signed  (2's comp)"  n_bits=coeff_prec  bin_pt=coeff_bp  dbl_ovrd=off  optimize=Area  use_rpm=off  block_type=sprom
      settings: xl_area=[7 14 0 14 0 0 0]  block_version=10.1
  ROM 7 : xbsIndex_r4/ROM  depth=polyphaseBranches  initVector=h(7*subFilterLength+1:8*subFilterLength)  distributed_mem=Distributed memory  rst=off  init_reg=0  en=off  latency=1  arith_type="Signed  (2's comp)"  n_bits=coeff_prec  bin_pt=coeff_bp  dbl_ovrd=off  optimize=Area  use_rpm=off  block_type=sprom
      settings: xl_area=[7 14 0 14 0 0 0]  block_version=10.1
  Register : xbsIndex_r4/Register  init=0  rst=off  en=on  dbl_ovrd=off  block_type=register
      settings: xl_area=[8 16 0 0 0 0 0]  block_version=10.1
  Relational : xbsIndex_r4/Relational  mode=a=b  en=off  latency=0  dbl_ovrd=off  block_type=relational
      settings: xl_area=[1 0 0 2 0 0 0]  block_version=10.1
  Time Division Demultiplexer : xbsIndex_r4/Time Division Demultiplexer  frame_pattern=ones(1,8)  impl_style=Multiple Channel  vin=off  dbl_ovrd=off  explicit_period=off  period=1  block_type=tdd
      settings: infoedit=Samples presented at the input are selected and down-sampled according to the frame sampling pattern specified. The sampled input is presented either as a single or multiple channel at the output.  xl_area=[135 270 0 0 0 0 0]  block_version=10.1
  Y : Outport
  wires:
  3-bit Counter/1 -> ROM 6/1, ROM 7/1, ROM 5/1, ROM 4/1, ROM 3/1, ROM 2/1, ROM 1/1, ROM 0/1, Relational/2, ASR 7/2, ASR 6/2, ASR 5/2, ASR 4/2, ASR 3/2, ASR 2/2, ASR 0/2, ASR 1/2
  ASR 7/1 -> Delay/1
  ASR 6/1 -> Delay1/1
  ASR 5/1 -> Delay2/1
  ASR 4/1 -> Delay3/1
  ASR 3/1 -> Delay4/1
  ASR 2/1 -> Delay5/1
  ASR 1/1 -> Delay6/1
  ASR 0/1 -> Delay7/1
  Mult8/1 -> Adder Tree/8(In8)
  Mult6/1 -> Adder Tree/7(In7)
  Mult5/1 -> Adder Tree/6(In6)
  Mult4/1 -> Adder Tree/5(In5)
  Mult3/1 -> Adder Tree/4(In4)
  Mult2/1 -> Adder Tree/3(In3)
  Mult1/1 -> Adder Tree/2(In2)
  Mult/1 -> Adder Tree/1(In1)
  ROM 0/1 -> Mult8/2
  ROM 1/1 -> Mult6/2
  ROM 2/1 -> Mult5/2
  ROM 3/1 -> Mult4/2
  ROM 4/1 -> Mult3/2
  ROM 5/1 -> Mult2/2
  ROM 6/1 -> Mult1/2
  ROM 7/1 -> Mult/2
  Accumulator/1 -> Register/1
  Constant/1 -> Relational/1
  Relational/1 -> Accumulator/2, Register/2
  Down Sample/1 -> Y/1
  Register/1 -> Down Sample/1
  Adder Tree/1(Out1) -> Accumulator/1
  X/1 -> Time Division Demultiplexer/1
  Time Division Demultiplexer/1 -> ASR 0/1
  Time Division Demultiplexer/2 -> ASR 1/1
  Time Division Demultiplexer/3 -> ASR 2/1
  Time Division Demultiplexer/4 -> ASR 3/1
  Time Division Demultiplexer/5 -> ASR 4/1
  Time Division Demultiplexer/6 -> ASR 5/1
  Time Division Demultiplexer/7 -> ASR 6/1
  Time Division Demultiplexer/8 -> ASR 7/1
  Delay/1 -> Mult8/1
  Delay1/1 -> Mult6/1
  Delay2/1 -> Mult5/1
  Delay3/1 -> Mult4/1
  Delay4/1 -> Mult3/1
  Delay5/1 -> Mult2/1
  Delay6/1 -> Mult1/1
  Delay7/1 -> Mult/1

== system simple_streaming_txrx/Receiver/Downconverter/ComplexMult ==
  A I : Inport
  A Q : Inport  Port=2
  B I : Inport  Port=3
  B Q : Inport  Port=4
  AddSub : xbsIndex_r4/AddSub  mode=Subtraction  use_carryin=off  use_carryout=off  en=off  latency=0  precision=User Defined  arith_type="Signed  (2's comp)"  n_bits=18  bin_pt=17  quantization=Truncate  overflow=Wrap  dbl_ovrd=off  use_behavioral_HDL=off  pipelined=off  use_rpm=on  block_type=addsub
      settings: xl_area=[9 0 0 18 0 0 0]  block_version=10.1
  AddSub1 : xbsIndex_r4/AddSub  mode=Addition  use_carryin=off  use_carryout=off  en=off  latency=0  precision=User Defined  arith_type="Signed  (2's comp)"  n_bits=18  bin_pt=17  quantization=Truncate  overflow=Wrap  dbl_ovrd=off  use_behavioral_HDL=off  pipelined=off  use_rpm=on  block_type=addsub
      settings: xl_area=[9 0 0 18 0 0 0]  block_version=10.1
  Mult{,1..3} (4 alike) : xbsIndex_r4/Mult  precision=User Defined  arith_type="Signed  (2's comp)"  n_bits=18  bin_pt=17  quantization=Truncate  overflow=Wrap  en=off  latency=1  dbl_ovrd=off  use_behavioral_HDL=off  use_embedded=on  opt=Speed  optimum_pipeline=off  pipeline=on  use_rpm=on  placement_style=Triangular  block_type=mult
      settings: infoedit=Hardware notes: To use the internal pipeline stage of the dedicated multiplier you must select 'Pipeline for maximum performance'.  xl_area=[9 -11 0 18 0 1 0]  block_version=10.1
  I : Outport
  Q : Outport  Port=2
  wires:
  Mult/1 -> AddSub/1
  Mult1/1 -> AddSub/2
  Mult2/1 -> AddSub1/1
  Mult3/1 -> AddSub1/2
  AddSub/1 -> I/1
  AddSub1/1 -> Q/1
  A I/1 -> Mult/1, Mult3/1
  B I/1 -> Mult/2, Mult2/2
  A Q/1 -> Mult1/1, Mult2/1
  B Q/1 -> Mult1/2, Mult3/2

== system simple_streaming_txrx/Receiver/Downconverter/myDDS ==
  phase inc : Inport
  10MSB : xbsIndex_r4/Slice  nbits=10  boolean_output=off  mode=Upper Bit Location + Width  bit1=0  base1=MSB of Input  bit0=0  base0=LSB of Input  dbl_ovrd=off  block_type=slice
      settings: infoedit="Extracts a given range of bits from each input sample and presents it at the output.  The output type is ordinarily unsigned with binary point at zero, but can be Boolean when the slice is one bit wide.<P><P>Hardware notes: In hardware this block costs nothing."  block_version=10.1
  Accumulator : xbsIndex_r4/Accumulator  operation=Add  n_bits=32  overflow=Wrap  scale=1  rst=off  hasbypass=off  en=off  dbl_ovrd=off  use_behavioral_HDL=on  block_type=accum
      settings: infoedit="Adder or subtractor-based accumulator.   Output type and binary point position match the input.<P><P>Hardware notes: When \"Reinitialize with input 'b' on reset\" is selected, the accumulator is forced to run at the system rate even if the input 'b' is running at a slower rate."  xl_area=[16 32 0 32 0 0 0]  block_version=10.1
  Cos ROM : xbsIndex_r4/ROM  depth=1024  initVector=cos(2*pi*[0:1023]/1024)  distributed_mem=Block RAM  rst=off  init_reg=0  en=off  latency=1  arith_type="Signed  (2's comp)"  n_bits=16  bin_pt=15  dbl_ovrd=off  optimize=Area  use_rpm=off  block_type=sprom
      settings: xl_area=[0 0 1 0 0 0 0]  block_version=10.1
  Sin ROM : xbsIndex_r4/ROM  depth=1024  initVector=sin(2*pi*[0:1023]/1024)  distributed_mem=Block RAM  rst=off  init_reg=0  en=off  latency=1  arith_type="Signed  (2's comp)"  n_bits=16  bin_pt=15  dbl_ovrd=off  optimize=Area  use_rpm=off  block_type=sprom
      settings: xl_area=[0 0 1 0 0 0 0]  block_version=10.1
  sin : Outport
  cos : Outport  Port=2
  wires:
  Accumulator/1 -> 10MSB/1
  phase inc/1 -> Accumulator/1
  Cos ROM/1 -> cos/1
  Sin ROM/1 -> sin/1
  10MSB/1 -> Cos ROM/1, Sin ROM/1

== system simple_streaming_txrx/Receiver/Timing Recovery/2nd Order Filter ==
  Err In : Inport
  Reset : Inport  Port=2
  AddSub1 : xbsIndex_r4/AddSub  mode=Addition  use_carryin=off  use_carryout=off  en=off  latency=0  precision=Full  arith_type="Signed  (2's comp)"  n_bits=8  bin_pt=2  quantization=Truncate  overflow=Flag as error  dbl_ovrd=off  use_behavioral_HDL=on  pipelined=off  use_rpm=on  block_type=addsub
      settings: xl_area=[17 0 0 33 0 0 0]  block_version=10.1
  AddSub2 : xbsIndex_r4/AddSub  mode=Addition  use_carryin=off  use_carryout=off  en=off  latency=0  precision=User Defined  arith_type="Signed  (2's comp)"  n_bits=35  bin_pt=34  quantization=Truncate  overflow=Flag as error  dbl_ovrd=off  use_behavioral_HDL=on  pipelined=off  use_rpm=on  block_type=addsub
      settings: xl_area=[17 0 0 33 0 0 0]  block_version=10.1
  Delay1 : xbsIndex_r4/Delay  en=off  latency=1  dbl_ovrd=off  reg_retiming=off  block_type=delay
      settings: xl_area=[18 35 0 0 0 0 0]  block_version=10.1
  Delay2 : xbsIndex_r4/Delay  en=off  latency=1  dbl_ovrd=off  reg_retiming=off  block_type=delay
      settings: xl_area=[16 32 0 0 0 0 0]  block_version=10.1
  Display : Display
  Display1 : Display
  Gateway Out{,1..3} (4 alike) : xbsIndex_r4/Gateway Out  hdl_port=off  timing_constraint=None  locs_specified=off  LOCs={}  block_type=gatewayout
      settings: infoedit="Gateway out block.  Converts Xilinx fixed point inputs into ouputs of type Simulink integer, double, or fixed point.<P><P>Hardware notes:  In hardware these blocks become top level output ports or are discarded, depending on how they are configured."  xl_area=[0 0 0 0 0 0 0]  block_version=10.1
  Mult1 : xbsIndex_r4/Mult  precision=User Defined  arith_type="Signed  (2's comp)"  n_bits=32  bin_pt=31  quantization=Truncate  overflow=Flag as error  en=off  latency=3  dbl_ovrd=off  use_behavioral_HDL=off  use_embedded=on  opt=Speed  optimum_pipeline=off  pipeline=on  use_rpm=on  placement_style=Rectangular shape  block_type=mult
      settings: infoedit=Hardware notes: To use the internal pipeline stage of the dedicated multiplier you must select 'Pipeline for maximum performance'.  xl_area=[41 81 0 81 0 2 0]  block_version=10.1
  Mult2 : xbsIndex_r4/Mult  precision=User Defined  arith_type="Signed  (2's comp)"  n_bits=32  bin_pt=31  quantization=Truncate  overflow=Flag as error  en=off  latency=3  dbl_ovrd=off  use_behavioral_HDL=off  use_embedded=on  opt=Speed  optimum_pipeline=off  pipeline=on  use_rpm=on  placement_style=Rectangular shape  block_type=mult
      settings: infoedit=Hardware notes: To use the internal pipeline stage of the dedicated multiplier you must select 'Pipeline for maximum performance'.  xl_area=[41 81 0 81 0 2 0]  block_version=10.1
  Mult3 : xbsIndex_r4/Mult  precision=User Defined  arith_type="Signed  (2's comp)"  n_bits=32  bin_pt=31  quantization=Truncate  overflow=Wrap  en=off  latency=3  dbl_ovrd=off  use_behavioral_HDL=off  use_embedded=on  opt=Speed  optimum_pipeline=off  pipeline=on  use_rpm=on  placement_style=Rectangular shape  block_type=mult
      settings: infoedit=Hardware notes: To use the internal pipeline stage of the dedicated multiplier you must select 'Pipeline for maximum performance'.  xl_area=[65 112 0 112 0 3 0]  block_version=10.1
  Register1 : xbsIndex_r4/Register  init=0  rst=on  en=off  dbl_ovrd=off  block_type=register
      settings: xl_area=[18 36 0 0 0 0 0]  block_version=10.1
  Register2 : xbsIndex_r4/Register  Orientation=left  init=0  rst=on  en=off  dbl_ovrd=off  block_type=register
      settings: xl_area=[18 35 0 0 0 0 0]  block_version=10.1
  Scope : Scope  NumInputPorts=2
      settings: YMin=0.0002125~-0.000256348  YMax=0.000245~-0.000231934  SaveName=ScopeData2
  Err Filt : Outport
  wires:
  Delay2/1 -> AddSub1/1, Gateway Out2/1
  Register2/1 -> AddSub2/2
  AddSub2/1 -> Delay1/1, Gateway Out3/1, Register2/1
  Mult1/1 -> AddSub2/1
  Mult2/1 -> Delay2/1
  AddSub1/1 -> Register1/1
  Reset/1 -> Register1/2, Register2/2
  Err In/1 -> Mult2/2, Mult1/1
  [TIMING_KI] -> Mult1/2, Gateway Out1/1
  [TIMING_KP] -> Mult2/1, Gateway Out/1
  Delay1/1 -> AddSub1/2
  Gateway Out/1 -> Display/1
  Gateway Out1/1 -> Display1/1
  Gateway Out2/1 -> Scope/1
  Gateway Out3/1 -> Scope/2
  [TIMING_K] -> Mult3/1
  Register1/1 -> Mult3/2
  Mult3/1 -> Err Filt/1

== system simple_streaming_txrx/Receiver/Timing Recovery/Timing Error Detector ==
  dI : Inport
  I : Inport  Port=2
  Accumulator : xbsIndex_r4/Accumulator  operation=Add  n_bits=24  overflow=Wrap  scale=1  rst=off  hasbypass=off  en=off  dbl_ovrd=off  use_behavioral_HDL=on  block_type=accum
      settings: infoedit="Adder or subtractor-based accumulator.   Output type and binary point position match the input.<P><P>Hardware notes: When \"Reinitialize with input 'b' on reset\" is selected, the accumulator is forced to run at the system rate even if the input 'b' is running at a slower rate."  xl_area=[12 24 0 24 0 0 0]  block_version=10.1
  AddSub : xbsIndex_r4/AddSub  mode=Subtraction  use_carryin=off  use_carryout=off  en=off  latency=0  precision=Full  arith_type=Unsigned  n_bits=8  bin_pt=2  quantization=Truncate  overflow=Wrap  dbl_ovrd=off  use_behavioral_HDL=on  pipelined=off  use_rpm=on  block_type=addsub
      settings: xl_area=[9 0 0 17 0 0 0]  block_version=10.1
  Delay : xbsIndex_r4/Delay  en=off  latency=8  dbl_ovrd=off  reg_retiming=off  block_type=delay
      settings: xl_area=[8 16 0 16 0 0 0]  block_version=10.1
  Mult : xbsIndex_r4/Mult  precision=User Defined  arith_type="Signed  (2's comp)"  n_bits=16  bin_pt=14  quantization=Truncate  overflow=Wrap  en=off  latency=1  dbl_ovrd=off  use_behavioral_HDL=off  use_embedded=on  opt=Speed  optimum_pipeline=off  pipeline=on  use_rpm=on  placement_style=Rectangular shape  block_type=mult
      settings: infoedit=Hardware notes: To use the internal pipeline stage of the dedicated multiplier you must select 'Pipeline for maximum performance'.  xl_area=[8 -1 0 16 0 1 0]  block_version=10.1
  Scale : xbsIndex_r4/Scale  scale_factor=-3  dbl_ovrd=off  block_type=scale
      settings: infoedit=Scales input by a power of two by adjusting the binary point position.<P><P>Hardware notes: In hardware this block costs nothing.  block_version=10.1
  Threshold : xbsIndex_r4/Threshold  en=off  latency=0  dbl_ovrd=off  block_type=sgn
      settings: infoedit="Presents -1 as output if input is negative; otherwise presents 1.  Output is a two bit signed number."  xl_area=[0 0 0 0 0 0 0]  block_version=10.1
  Err : Outport
  wires:
  Threshold/1 -> Mult/1
  I/1 -> Threshold/1
  dI/1 -> Mult/2
  Delay/1 -> AddSub/2
  AddSub/1 -> Accumulator/1
  Accumulator/1 -> Scale/1
  Mult/1 -> AddSub/1, Delay/1, Err/1
